simulink model "eskf16_block"  (R2025b)
settings: Solver=FixedStepDiscrete  StartTime=0.0  StopTime=5  FixedStep=2e-3  RelTol=1e-3
settings Model: Creator=Ashwin  LastModifiedBy=Ashwin

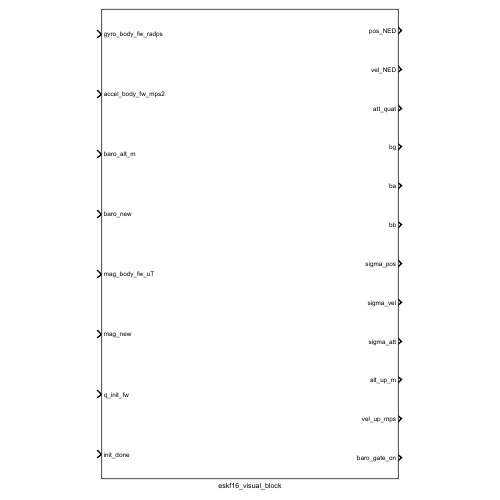
[thumbnail: Simulink's stored preview of the top-level diagram]
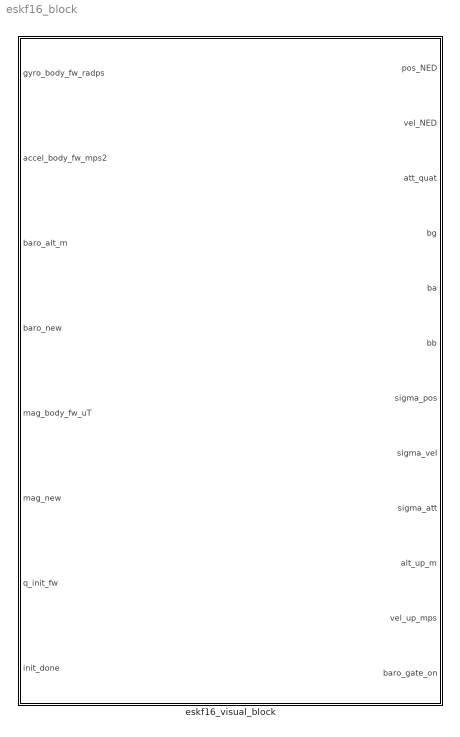
== system eskf16_block ==
  eskf16_visual_block : Subsystem

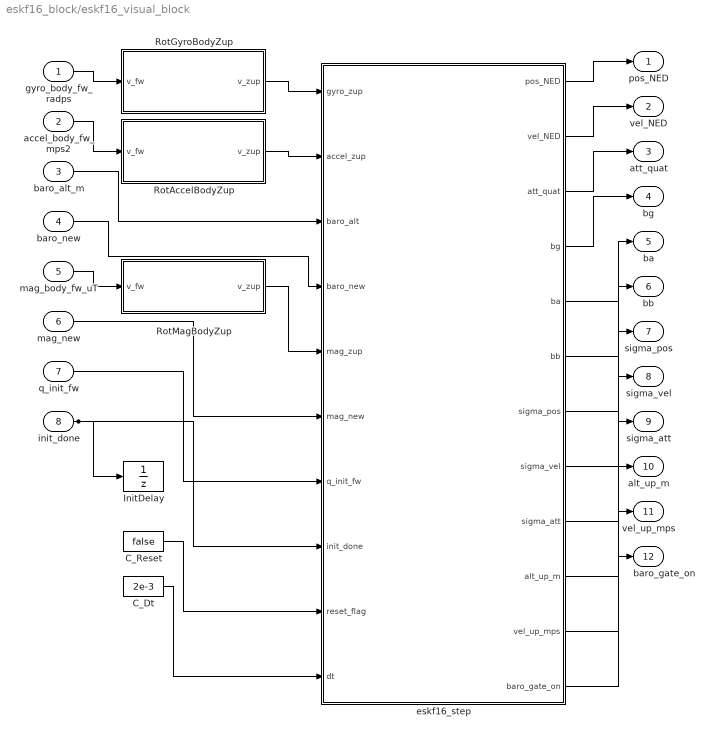
== system eskf16_block/eskf16_visual_block ==
  gyro_body_fw_radps : Inport
  accel_body_fw_mps2 : Inport  Port=2
  baro_alt_m : Inport  Port=3
  baro_new : Inport  Port=4
  mag_body_fw_uT : Inport  Port=5
  mag_new : Inport  Port=6
  q_init_fw : Inport  Port=7
  init_done : Inport  Port=8
  C_Dt : Constant  Value=2e-3  SampleTime=-1
  C_Reset : Constant  Value=false  OutDataTypeStr=boolean  SampleTime=-1
  InitDelay : UnitDelay  SampleTime=-1  HasFrameUpgradeWarning=on
  RotAccelBodyZup : MATLAB Function  TreatAsAtomicUnit=on
  RotGyroBodyZup : MATLAB Function  TreatAsAtomicUnit=on
  RotMagBodyZup : MATLAB Function  TreatAsAtomicUnit=on
  eskf16_step : MATLAB Function  TreatAsAtomicUnit=on
  pos_NED : Outport
  vel_NED : Outport  Port=2
  att_quat : Outport  Port=3
  bg : Outport  Port=4
  ba : Outport  Port=5
  bb : Outport  Port=6
  sigma_pos : Outport  Port=7
  sigma_vel : Outport  Port=8
  sigma_att : Outport  Port=9
  alt_up_m : Outport  Port=10
  vel_up_mps : Outport  Port=11
  baro_gate_on : Outport  Port=12
  wires:
  gyro_body_fw_radps/1 -> RotGyroBodyZup/1(v_fw)
  accel_body_fw_mps2/1 -> RotAccelBodyZup/1(v_fw)
  mag_body_fw_uT/1 -> RotMagBodyZup/1(v_fw)
  init_done/1 -> InitDelay/1, eskf16_step/8(init_done)
  RotGyroBodyZup/1(v_zup) -> eskf16_step/1(gyro_zup)
  RotAccelBodyZup/1(v_zup) -> eskf16_step/2(accel_zup)
  baro_alt_m/1 -> eskf16_step/3(baro_alt)
  baro_new/1 -> eskf16_step/4(baro_new)
  RotMagBodyZup/1(v_zup) -> eskf16_step/5(mag_zup)
  mag_new/1 -> eskf16_step/6(mag_new)
  q_init_fw/1 -> eskf16_step/7(q_init_fw)
  C_Reset/1 -> eskf16_step/9(reset_flag)
  C_Dt/1 -> eskf16_step/10(dt)
  eskf16_step/1(pos_NED) -> pos_NED/1
  eskf16_step/2(vel_NED) -> vel_NED/1
  eskf16_step/3(att_quat) -> att_quat/1
  eskf16_step/4(bg) -> bg/1
  eskf16_step/5(ba) -> ba/1
  eskf16_step/6(bb) -> bb/1
  eskf16_step/7(sigma_pos) -> sigma_pos/1
  eskf16_step/8(sigma_vel) -> sigma_vel/1
  eskf16_step/9(sigma_att) -> sigma_att/1
  eskf16_step/10(alt_up_m) -> alt_up_m/1
  eskf16_step/11(vel_up_mps) -> vel_up_mps/1
  eskf16_step/12(baro_gate_on) -> baro_gate_on/1

== matlab function eskf16_block/eskf16_visual_block/RotAccelBodyZup ==
  data: v_fw input; v_zup output
function v_zup = fcn(v_fw)
%#codegen
v = double(v_fw(:));
v_zup = [ v(1);  -v(3);  v(2) ];
end

== matlab function eskf16_block/eskf16_visual_block/RotGyroBodyZup ==
  data: v_fw input; v_zup output
function v_zup = fcn(v_fw)
%#codegen
v = double(v_fw(:));
v_zup = [ v(1);  -v(3);  v(2) ];
end

== matlab function eskf16_block/eskf16_visual_block/RotMagBodyZup ==
  data: v_fw input; v_zup output
function v_zup = fcn(v_fw)
%#codegen
v = double(v_fw(:));
v_zup = [ v(1);  -v(3);  v(2) ];
end

== matlab function eskf16_block/eskf16_visual_block/eskf16_step ==
  data: gyro_zup input; pos_NED output; accel_zup input; baro_alt input; baro_new input; mag_zup input; mag_new input; q_init_fw input; init_done input; reset_flag input; dt input; vel_NED output; att_quat output; bg output; ba output; bb output; sigma_pos output; sigma_vel output; sigma_att output; alt_up_m output; vel_up_mps output; baro_gate_on output
function [pos_NED, vel_NED, att_quat, bg, ba, bb, sigma_pos, sigma_vel, sigma_att, alt_up_m, vel_up_mps, baro_gate_on] = fcn(gyro_zup, accel_zup, baro_alt, baro_new, mag_zup, mag_new, q_init_fw, init_done, reset_flag, dt)
%#codegen
coder.extrinsic('casper_eskf16_helper');
pos_NED      = zeros(3,1);
vel_NED      = zeros(3,1);
att_quat     = [0;0;1;0];
bg           = zeros(3,1);
ba           = zeros(3,1);
bb           = double(0);
sigma_pos    = zeros(3,1);
sigma_vel    = zeros(3,1);
sigma_att    = zeros(3,1);
alt_up_m     = double(0);
vel_up_mps   = double(0);
baro_gate_on = false;
baro_innov_unused = double(0);
init_armed_unused = false;
[pos_NED, vel_NED, att_quat, bg, ba, bb, sigma_pos, sigma_vel, sigma_att, baro_gate_on, baro_innov_unused, init_armed_unused] = casper_eskf16_helper(double(gyro_zup), double(accel_zup), double(baro_alt), logical(baro_new), double(mag_zup), logical(mag_new), double(q_init_fw), logical(init_done), logical(reset_flag), double(dt));
alt_up_m   = -double(pos_NED(3));
vel_up_mps = -double(vel_NED(3));
end
